simulink subsystem "car"  (R2026a)
settings: Solver=VariableStepAuto
undefined symbols (not defined in the file): Free, Init, Vehicle, Visual, X, Y, Z
libraries: sm_lib x6, nesl_utility x4
settings Model: Creator=th12-dv  LastModifiedBy=th12-dv

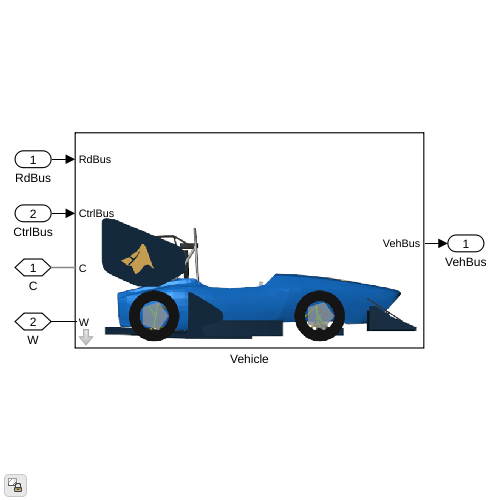
[thumbnail: Simulink's stored preview of the top-level diagram]
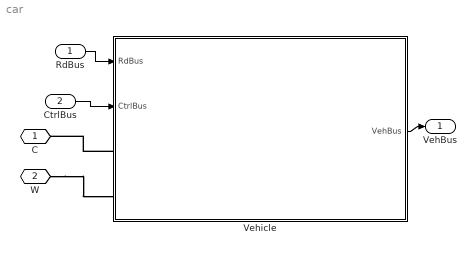
== system car ==
  RdBus : Inport
  CtrlBus : Inport  Port=2
  Vehicle : Subsystem  Tag=PublishSubsystem  VariantControl=NS_Con  mask(Vehicle with Two Axles){popup_BodyToWorld=Free, Vehicle=Vehicle, Init=Init, SpecifyPosTarget=on, veh_index=1, mask_image_name=sm_car_vehicle_hamba_IMAGE.png, Chassis=Vehicle.Chassis}
      mask prompts: popup_BodyToWorld "Body To World Connection"; Vehicle "Vehicle Parameters"; Init "Initial Values"; SpecifyPosTarget "Specify Position Target"; veh_index "Vehicle Index (for tires)"; mask_image_name "Mask Image (string)"
      mask help: Vehicle model with multibody suspension. Initial Values data structure sets initial speed of vehicle and wheels. Set tire index to ensure tire results can be saved independently from other vehicles in the model.
      mask Help: web('sm_car_doc_vehicle.html')
      mask TypeOptions popup_BodyToWorld: Body to World/popup_BodyToWorld
      mask TypeOptions SpecifyPosTarget: Body to World/SpecifyPosTarget
      mask TypeOptions veh_index: Chassis/veh_index
      mask DialogControl cont_sim Prompt: Config
      mask DialogControl cont_connections Prompt: Lock for KnC Test
      mask Display:
      | % Get image from BodyGeometry.class
      | % (active choice for Body Geometry subsystem)
      | temp_veh_bg_class = lower(get_param([gcb '/Chassis/Body/Body Geometry'],'LabelModeActiveChoice'));
      | 
      | imagestr = (['sm_car_vehicle_' temp_veh_bg_class '.png']);
      | if(~exist(imagestr))
      |     imagestr = ['sm_car_vehicle_axle2_default.png'];
      | end
      | 
      | image(imagestr);
  C : PMIOPort  Side=Left
  W : PMIOPort  Port=2  Side=Left
  VehBus : Outport  VectorParamsAs1DForOutWhenUnconnected=off
  wires:
  CtrlBus/1 -> Vehicle/2(CtrlBus)
  Vehicle/1(VehBus) -> VehBus/1
  RdBus/1 -> Vehicle/1(RdBus)
  connections:
  Vehicle/LConn1 -- C/RConn1
  W/RConn1 -- Vehicle/LConn2

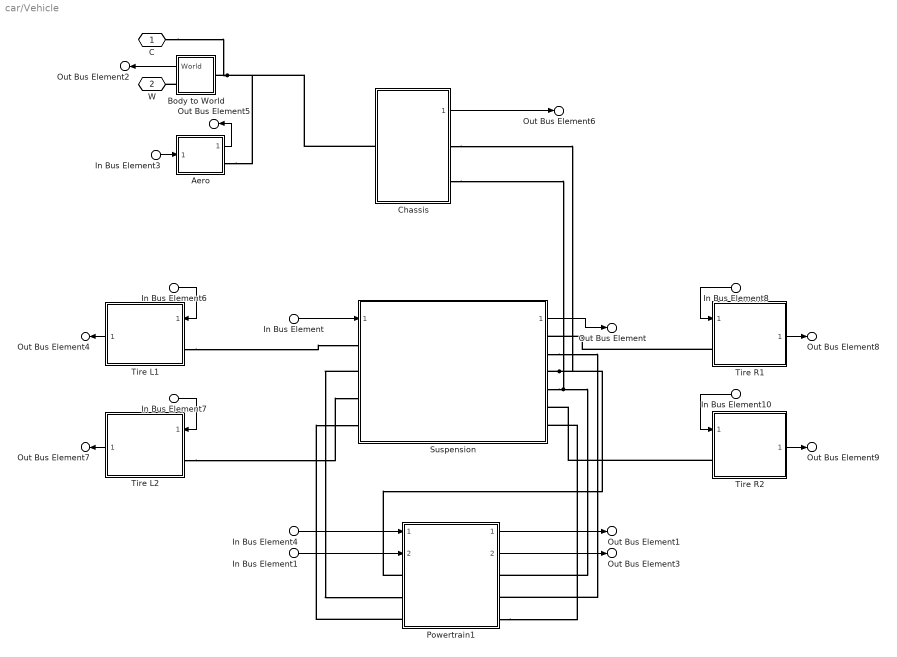
== system car/Vehicle ==
  In Bus Element3 : Inport  PortName=RdBus  Element=fWindCar
  In Bus Element6 : Inport  PortName=RdBus  Element=L1
  In Bus Element7 : Inport  PortName=RdBus  Element=L2
  In Bus Element8 : Inport  PortName=RdBus  Element=R1
  In Bus Element10 : Inport  PortName=RdBus  Element=R2
  In Bus Element : Inport  Port=2  PortName=CtrlBus  Element=Chassis
  In Bus Element1 : Inport  Port=2  PortName=CtrlBus  Element=Power
  In Bus Element4 : Inport  Port=2  PortName=CtrlBus  Element=Driveline
  Aero : Subsystem  mask(Aerodynamic Load (Drag, Lift)){CL=Chassis.Aero.CL.Value, CD=Chassis.Aero.CD.Value, rho=Chassis.Aero.rho_air.Value, A=Chassis.Aero.ARef.Value, sCentreOfPressure=Chassis.Aero.sPressureCentre.Value, clr_hp=Visual.hp.clr, opc_hp=Visual.hp.opc, rad_hp=Visual.hp.rad}
      mask prompts: CL "Lift Coeff (-)"; CD "Drag Coeff (-)"; rho "Air Density (kg/m^3)"; A "Reference Area (m^2)"; sCentreOfPressure "Centre of Pressure [xyz] (m)"; clr_hp "Color [RGB]"; opc_hp "Opacity (0-1)"; rad_hp "Radius (m)"
      mask help: Models lift and drag on vehicle.
      mask TypeOptions clr_hp:
      | Vis
      | Center of Pressure/GraphicDiffuseColor
      mask TypeOptions opc_hp:
      | Vis
      | Center of Pressure/GraphicOpacity
      mask TypeOptions rad_hp:
      | Vis
      | Center of Pressure/SphereRadius
      mask DialogControl conv_vis Prompt: Visualization
  Body to World : Subsystem  Variant=on  VariantControlMode=label  VariantControl=Choice  LabelModeActiveChoice=Free  mask{popup_BodyToWorld=Free, SpecifyPosTarget=on}
      mask prompts: popup_BodyToWorld "Body To World Connection"; SpecifyPosTarget "Specify Position Target"
      mask init:
      | bh = gcb;
      | b2w = get_param(bh,'popup_BodyToWorld');
      | set_param(bh,'LabelModeActiveChoice',b2w)
      | if(strcmp(b2w,'Free'))
      |     set_param([bh '/Free'],'SpecifyPosTarget',get_param(bh,'SpecifyPosTarget'));
      | end
      mask TypeOptions popup_BodyToWorld: Free | Rigid
      mask Display: disp(' ')
  Chassis : Subsystem  ReferencedSubsystem=th11_Chassis  Chassis=Vehicle.Chassis  Init=Init  mask_image_name=sm_car_vehicle_chassis_hamba_IMAGE.png  veh_index=veh_index  hp_mount_a1=Chassis.Body.sAxle1.Value  hp_mount_a2=Chassis.Body.sAxle2.Value  hp_chassis_cg=Chassis.Body.sCG.Value  chassis_mass=Chassis.Body.m.Value  chassis_inertia=Chassis.Body.J.Value  BodyGeometry=Chassis.Body.BodyGeometry  clr_chassis_hp_cg=Visual.hp.clr  opc_chassis_hp_cg=Visual.hp.opc  size_chassis_hp_cg=Visual.hp.rad
  Powertrain1 : Subsystem  ReferencedSubsystem=th11_Powertrain  Powertrain=Vehicle.Powertrain
  Suspension : Subsystem  ReferencedSubsystem=th11_Suspension
  Tire L1 : Subsystem  ReferencedSubsystem=th11_Tire  popup_leftRight=Left  tir_index=veh_index  Tire=Chassis.TireA1  VariantLabel=Chassis.TireA1.class.Value
  Tire L2 : Subsystem  ReferencedSubsystem=th11_Tire  popup_leftRight=Left  tir_index=veh_index+10  Tire=Chassis.TireA2  VariantLabel=Chassis.TireA2.class.Value
  Tire R1 : Subsystem  ReferencedSubsystem=th11_Tire  popup_leftRight=Right  tir_index=veh_index+4  Tire=Chassis.TireA1  VariantLabel=Chassis.TireA1.class.Value
  Tire R2 : Subsystem  ReferencedSubsystem=th11_Tire  popup_leftRight=Right  tir_index=veh_index+14  Tire=Chassis.TireA2  VariantLabel=Chassis.TireA2.class.Value
  C : PMIOPort  Side=Left
  W : PMIOPort  Port=2  Side=Left
  Out Bus Element2 : Outport  VectorParamsAs1DForOutWhenUnconnected=off  PortName=VehBus  Element=World
  Out Bus Element5 : Outport  VectorParamsAs1DForOutWhenUnconnected=off  PortName=VehBus  Element=Aero
  Out Bus Element4 : Outport  VectorParamsAs1DForOutWhenUnconnected=off  PortName=VehBus  Element=WhlL1
  Out Bus Element7 : Outport  VectorParamsAs1DForOutWhenUnconnected=off  PortName=VehBus  Element=WhlL2
  Out Bus Element6 : Outport  VectorParamsAs1DForOutWhenUnconnected=off  PortName=VehBus  Element=Body
  Out Bus Element : Outport  VectorParamsAs1DForOutWhenUnconnected=off  PortName=VehBus  Element=Susp
  Out Bus Element8 : Outport  VectorParamsAs1DForOutWhenUnconnected=off  PortName=VehBus  Element=WhlR1
  Out Bus Element9 : Outport  VectorParamsAs1DForOutWhenUnconnected=off  PortName=VehBus  Element=WhlR2
  Out Bus Element1 : Outport  VectorParamsAs1DForOutWhenUnconnected=off  PortName=VehBus  Element=Driveline
  Out Bus Element3 : Outport  VectorParamsAs1DForOutWhenUnconnected=off  PortName=VehBus  Element=Power
  wires:
  In Bus Element1/1 -> Powertrain1/2
  In Bus Element4/1 -> Powertrain1/1
  Powertrain1/2 -> Out Bus Element3/1
  Powertrain1/1 -> Out Bus Element1/1
  Tire R1/1 -> Out Bus Element8/1
  Tire L2/1 -> Out Bus Element7/1
  In Bus Element3/1 -> Aero/1(fWind)
  In Bus Element6/1 -> Tire L1/1
  In Bus Element10/1 -> Tire R2/1
  In Bus Element7/1 -> Tire L2/1
  In Bus Element8/1 -> Tire R1/1
  Tire R2/1 -> Out Bus Element9/1
  Chassis/1 -> Out Bus Element6/1
  Tire L1/1 -> Out Bus Element4/1
  Body to World/1(World) -> Out Bus Element2/1
  In Bus Element/1 -> Suspension/1
  Suspension/1 -> Out Bus Element/1
  Aero/1(meas) -> Out Bus Element5/1
  connections:
  Body to World/RConn1 -- W/RConn1
  Tire L2/LConn1 -- Suspension/LConn3
  Suspension/RConn2 -- Powertrain1/RConn2
  Chassis/RConn2 -- Powertrain1/RConn1 -- Suspension/RConn4
  Suspension/LConn2 -- Powertrain1/LConn2
  Powertrain1/RConn3 -- Suspension/RConn6
  Powertrain1/LConn3 -- Suspension/LConn4
  Chassis/LConn1 -- Aero/RConn1 -- C/RConn1 -- Body to World/LConn1
  Tire R1/LConn1 -- Suspension/RConn1
  Tire L1/LConn1 -- Suspension/LConn1
  Suspension/RConn3 -- Chassis/RConn1 -- Powertrain1/LConn1
  Tire R2/LConn1 -- Suspension/RConn5

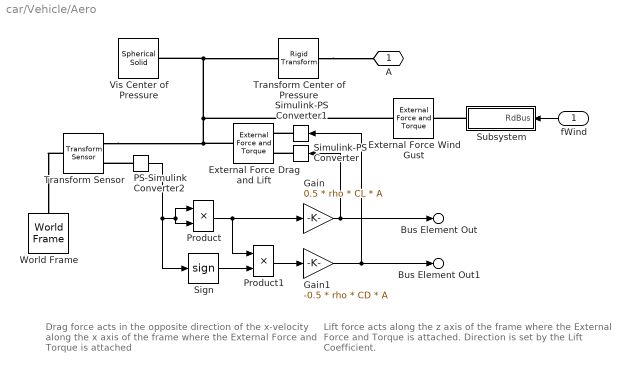
== system car/Vehicle/Aero ==
  note: Drag force acts in the opposite direction of the x-velocity along the x axis of the frame where the External Force and Torque is attached
  note: Lift force acts along the z axis of the frame where the External Force and Torque is attached. Direction is set by the Lift Coefficient.
  fWind : Inport
  External Force Drag and Lift : sm_lib/Forces and Torques/External Force and Torque  EnableForceX=on  EnableForceY=off  EnableForceZ=on  EnableForce=off  ForceResolutionFrame=AttachedFrame  EnableTorqueX=off  EnableTorqueY=off  EnableTorqueZ=off  EnableTorque=off  TorqueResolutionFrame=AttachedFrame
  External Force Wind Gust : sm_lib/Forces and Torques/External Force and Torque  EnableForceX=off  EnableForceY=off  EnableForceZ=off  EnableForce=on  ForceResolutionFrame=World  EnableTorqueX=off  EnableTorqueY=off  EnableTorqueZ=off  EnableTorque=off  TorqueResolutionFrame=AttachedFrame
  Gain : Gain  Gain=0.5 * rho * CL * A
  Gain1 : Gain  Gain=-0.5 * rho * CD * A
  PS-Simulink Converter2 : nesl_utility/PS-Simulink Converter  PhysicalDomain=network_engine_domain  SubClassName=ps_output  LeftPortType=input  RightPortType=output  PseudoPeriodic=off  Frequencies=[]  VectorFormat=1-D array  Unit=1  AffineConversion=off
  Product : Product
  Product1 : Product
  Sign : Signum  ZeroCross=off
  Simulink-PS Converter : nesl_utility/Simulink-PS Converter  PhysicalDomain=network_engine_domain  SubClassName=ps_input  LeftPortType=input  RightPortType=output  PseudoPeriodic=off  Frequencies=[]  NoiseDistribution=none  NoiseParameters=[]  Unit=1  AffineConversion=off  FilteringAndDerivatives=provide  SimscapeFilterOrder=1  InputFilterTimeConstant=0.001  UdotUserProvided=0
  Simulink-PS Converter1 : nesl_utility/Simulink-PS Converter  PhysicalDomain=network_engine_domain  SubClassName=ps_input  LeftPortType=input  RightPortType=output  PseudoPeriodic=off  Frequencies=[]  NoiseDistribution=none  NoiseParameters=[]  Unit=1  AffineConversion=off  FilteringAndDerivatives=provide  SimscapeFilterOrder=1  InputFilterTimeConstant=0.001  UdotUserProvided=0
  Subsystem : Subsystem
  Transform Center of Pressure : sm_lib/Frames and Transforms/Rigid Transform  RotationMethod=None  FollAlignAxisA=+X  BaseAlignAxisA=+Y  FollAlignAxisB=+Y  BaseAlignAxisB=+Z  RotationStandardAxis=+Z  RotationAngle=0.0  RotationAngleUnits=deg  RotationArbitraryAxis=[0 0 1]  RotationSequenceAxes=FollowerAxes  RotationSequence=XYX  RotationSequenceAngles=[0 0 0]  RotationSequenceAnglesUnits=deg  RotationMatrix=[1 0 0; 0 1 0; 0 0 1]  Quaternion=[1 0 0 0]  TranslationMethod=Cartesian  TranslationCartesianOffset=sCentreOfPressure  TranslationCartesianOffsetUnits=m  TranslationStandardAxis=+Z  TranslationStandardOffset=0  TranslationStandardOffsetUnits=m  TranslationROffset=0  TranslationROffsetUnits=m  TranslationThetaOffset=0  TranslationThetaOffsetUnits=deg  TranslationZOffset=0  TranslationZOffsetUnits=m
  Transform Sensor : sm_lib/Frames and Transforms/Transform Sensor  MeasurementFrame=NonRotatingFollower  RotationSequence=XYX  SenseAngle=off  SenseAxis=off  SenseQ=off  SenseR=off  SenseRotationSequence=off  SenseOmegaX=off  SenseOmegaY=off  SenseOmegaZ=off  SenseOmega=off  SenseQDot=off  SenseRDot=off  SenseRotationSequenceDot=off  SenseAlphaX=off  SenseAlphaY=off  SenseAlphaZ=off  SenseAlpha=off  SenseQDDot=off  SenseRDDot=off  SenseX=off  SenseY=off  SenseZ=off  SenseXYZ=off  SenseRad=off  SenseAzim=off  SenseDist=off  SenseInc=off  SenseXDot=on  SenseYDot=off  SenseZDot=off  SenseXYZDot=off  SenseRadDot=off  SenseAzimDot=off  SenseDistDot=off  SenseIncDot=off  SenseXDDot=off  SenseYDDot=off  SenseZDDot=off  SenseXYZDDot=off  SenseRadDDot=off  SenseAzimDDot=off  SenseDistDDot=off  SenseIncDDot=off
  Vis Center of Pressure : sm_lib/Body Elements/Spherical Solid  SphereRadius=rad_hp  SphereRadiusUnits=m  ExportEntireGeometry=off  InertiaType=CalculateFromGeometry  BasedOnType=Density  Density=1000  DensityUnits=kg/m^3  Mass=1  MassUnits=kg  CenterOfMass=[0 0 0]  CenterOfMassUnits=m  MomentsOfInertia=[1 1 1]  MomentsOfInertiaUnits=kg*m^2  ProductsOfInertia=[0 0 0]  ProductsOfInertiaUnits=kg*m^2  GraphicType=FromGeometry  MarkerShape=Sphere  MarkerSize=10  GraphicVisPropType=SimpleVisualProperties  GraphicDiffuseColor=clr_hp  GraphicOpacity=opc_hp  GraphicSpecularColor=[0.5 0.5 0.5 1.0]  GraphicAmbientColor=[0.15 0.15 0.15 1.0]  GraphicEmissiveColor=[0.0 0.0 0.0 1.0]  GraphicShininess=75  DoExposeReferenceFrame=on  SerializedFrames=<Frames/>
  World Frame : sm_lib/Frames and Transforms/World Frame
  A : PMIOPort  Side=Right
  Bus Element Out1 : Outport  VectorParamsAs1DForOutWhenUnconnected=off  PortName=meas  Element=Fx
  Bus Element Out : Outport  VectorParamsAs1DForOutWhenUnconnected=off  PortName=meas  Element=Fz
  wires:
  Gain1/1 -> Bus Element Out1/1, Simulink-PS Converter1/1
  Gain/1 -> Bus Element Out/1, Simulink-PS Converter/1
  fWind/1 -> Subsystem/1(RdBus)
  Sign/1 -> Product1/2
  Product/1 -> Product1/1, Gain/1
  Product1/1 -> Gain1/1
  PS-Simulink Converter2/1 -> Sign/1, Product/2, Product/1
  connections:
  Transform Sensor/LConn1 -- World Frame/RConn1
  PS-Simulink Converter2/LConn1 -- Transform Sensor/RConn2
  Transform Center of Pressure/LConn1 -- A/RConn1
  External Force Drag and Lift/RConn1 -- Transform Sensor/RConn1 -- External Force Wind Gust/RConn1 -- Vis Center of Pressure/RConn1 -- Transform Center of Pressure/RConn1
  Subsystem/RConn1 -- External Force Wind Gust/LConn1
  Simulink-PS Converter1/RConn1 -- External Force Drag and Lift/LConn1
  Simulink-PS Converter/RConn1 -- External Force Drag and Lift/LConn2

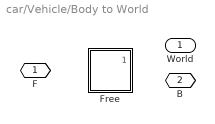
== system car/Vehicle/Body to World ==
  Free : Subsystem  VariantControl=Free  ReferencedSubsystem=th11_BodyToWorld_Free  Init=Init.Chassis  SpecifyPosTarget=on
  F : PMIOPort  Side=Left
  B : PMIOPort  Port=2  Side=Right
  World : Outport

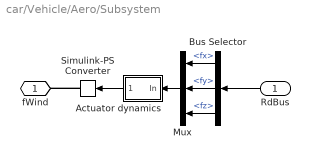
== system car/Vehicle/Aero/Subsystem ==
  RdBus : Inport
  Actuator dynamics : Subsystem  mask(First-order lag supporting vector signals){b=0.5, x_initial=0}
      mask prompts: b "Filter time constant"; x_initial "Initial output"
      mask help: Models a lag of the form 1/(b*s+1) where s is the Laplace operator.
  Bus Selector : BusSelector  OutputSignals=fx,fy,fz
  Mux : Mux  Inputs=3
  Simulink-PS Converter : nesl_utility/Simulink-PS Converter  PhysicalDomain=network_engine_domain  SubClassName=ps_input  LeftPortType=input  RightPortType=output  PseudoPeriodic=off  Frequencies=[]  NoiseDistribution=none  NoiseParameters=[]  Unit=1  AffineConversion=off  FilteringAndDerivatives=provide  SimscapeFilterOrder=1  InputFilterTimeConstant=0.001  UdotUserProvided=0
  fWind : PMIOPort  Side=Right
  wires:
  Mux/1 -> Actuator dynamics/1(In)
  Bus Selector/1 -> Mux/1  "<fx>"
  Bus Selector/2 -> Mux/2  "<fy>"
  Bus Selector/3 -> Mux/3  "<fz>"
  RdBus/1 -> Bus Selector/1
  Actuator dynamics/1(Out) -> Simulink-PS Converter/1
  connections:
  Simulink-PS Converter/RConn1 -- fWind/RConn1

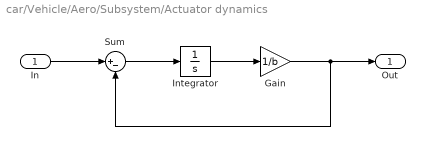
== system car/Vehicle/Aero/Subsystem/Actuator dynamics ==
  In : Inport
  Gain : Gain  Gain=1/b
  Integrator : Integrator  InitialCondition=x_initial*b
  Sum : Sum  Inputs=|+-  InputSameDT=on  SaturateOnIntegerOverflow=on  OutDataTypeStr=Inherit: Same as first input
  Out : Outport  VectorParamsAs1DForOutWhenUnconnected=off
  wires:
  Gain/1 -> Out/1, Sum/2
  Integrator/1 -> Gain/1
  In/1 -> Sum/1
  Sum/1 -> Integrator/1
